simulink model "projsim"  (R2016a)
settings: Solver=VariableStepAuto  StartTime=0.0  StopTime=t_end  MaxStep=1/(w_e*50)  RelTol=1e-3
values from neighbouring files (symbols this model uses):
  bw_tot = 0.2    [cod.m]
  Csr = (Ls*Lr)/((Ls*Lr)-M^2)    (= 22.6278248588)    [cod.m]
  H_tot = 1.6    [cod.m]
  K_i = 0    [cod.m]
  K_p = 1    [cod.m]
  kt_l = 0    [cod.m]
  Lr = M+.0008    (= 0.0358)    [cod.m]
  Ls = M+.0008    (= 0.0358)    [cod.m]
  M = .035    (= 0.035)    [cod.m]
  P = 4    [cod.m]
  Rr = .1    (= 0.1)    [cod.m]
  Rs = .1    (= 0.1)    [cod.m]
  V_bus = 500    [cod.m]
  w_e_command = 2*pi*60    (= 376.991118431)    [cod.m]
settings Model: Creator=JSD5266  LastModifiedBy=Seth Barger

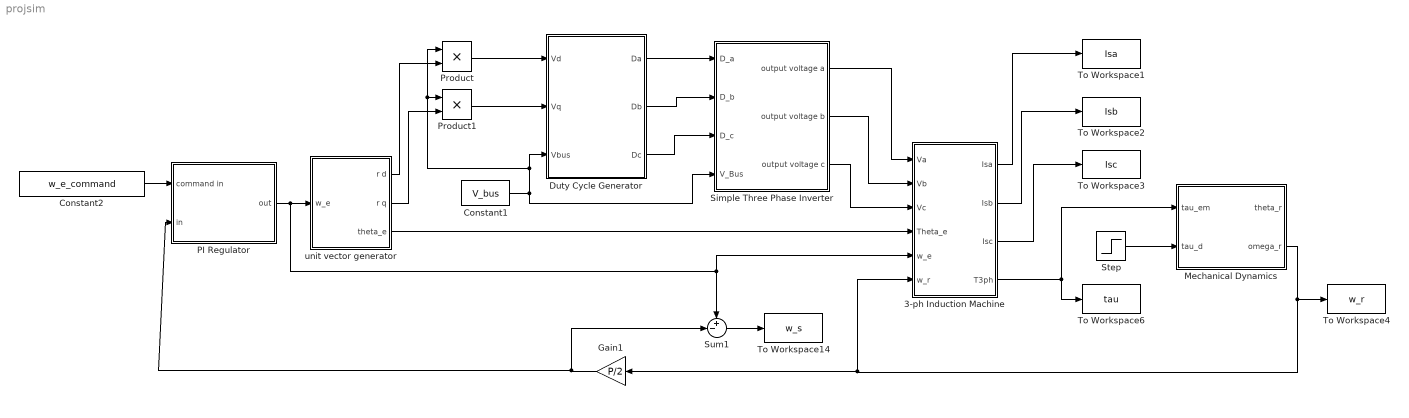
== system projsim ==
  3-ph Induction Machine : Subsystem
  Constant1 : Constant  Value=V_bus
  Constant2 : Constant  Value=w_e_command
  Duty Cycle Generator : Subsystem
  Gain1 : Gain  Gain=P/2
  Mechanical Dynamics : Subsystem
  PI Regulator : Subsystem
  Product : Product
  Product1 : Product
  Simple Three Phase Inverter : Subsystem
  Step : Step  Time=3  After=200  SampleTime=0
  Sum1 : Sum  Inputs=+-|
  To Workspace1 : ToWorkspace  VariableName=Isa  SampleTime=-1
  To Workspace14 : ToWorkspace  VariableName=w_s  SampleTime=-1
  To Workspace2 : ToWorkspace  VariableName=Isb  SampleTime=-1
  To Workspace3 : ToWorkspace  VariableName=Isc  SampleTime=-1
  To Workspace4 : ToWorkspace  VariableName=w_r  SampleTime=-1
  To Workspace6 : ToWorkspace  VariableName=tau  SampleTime=-1
  unit vector generator : Subsystem
  wires:
  3-ph Induction Machine/4(T3ph) -> To Workspace6/1, Mechanical Dynamics/1(tau_em)
  unit vector generator/3(theta_e) -> 3-ph Induction Machine/4(Theta_e)
  Step/1 -> Mechanical Dynamics/2(tau_d)
  Sum1/1 -> To Workspace14/1
  Gain1/1 -> PI Regulator/2(in), Sum1/2
  Simple Three Phase Inverter/3(output voltage c) -> 3-ph Induction Machine/3(Vc)
  Simple Three Phase Inverter/2(output voltage b) -> 3-ph Induction Machine/2(Vb)
  Simple Three Phase Inverter/1(output voltage a) -> 3-ph Induction Machine/1(Va)
  Duty Cycle Generator/1(Da) -> Simple Three Phase Inverter/1(D_a)
  Duty Cycle Generator/2(Db) -> Simple Three Phase Inverter/2(D_b)
  Duty Cycle Generator/3(Dc) -> Simple Three Phase Inverter/3(D_c)
  Constant1/1 -> Product1/1, Product/1, Duty Cycle Generator/3(Vbus), Simple Three Phase Inverter/4(V_Bus)
  Product/1 -> Duty Cycle Generator/1(Vd)
  unit vector generator/1(r d) -> Product/2
  Product1/1 -> Duty Cycle Generator/2(Vq)
  unit vector generator/2(r q) -> Product1/2
  Mechanical Dynamics/2(omega_r) -> To Workspace4/1, 3-ph Induction Machine/6(w_r), Gain1/1
  PI Regulator/1(out) -> Sum1/1, 3-ph Induction Machine/5(w_e), unit vector generator/1(w_e)
  Constant2/1 -> PI Regulator/1(command in)
  3-ph Induction Machine/1(Isa) -> To Workspace1/1
  3-ph Induction Machine/2(Isb) -> To Workspace2/1
  3-ph Induction Machine/3(Isc) -> To Workspace3/1

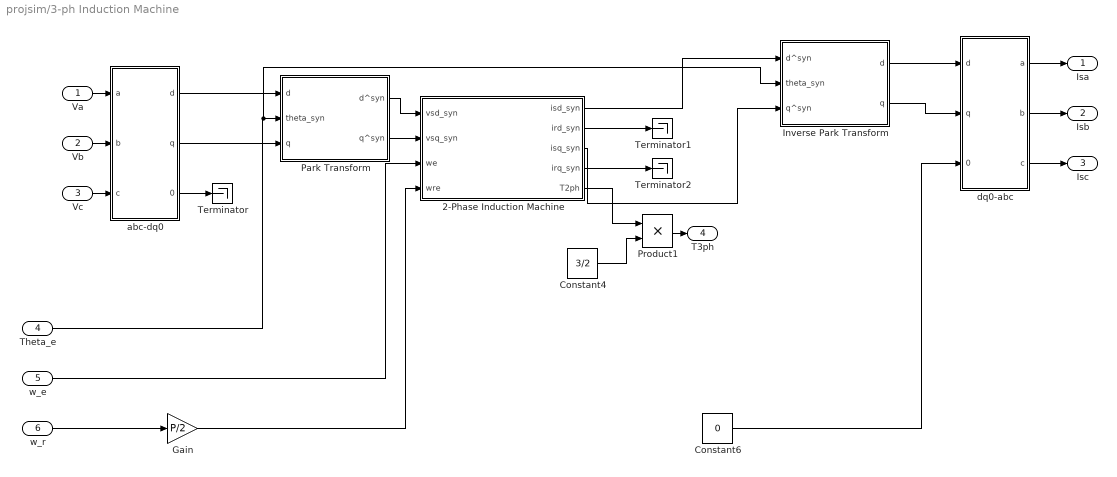
== system projsim/3-ph Induction Machine ==
  Va : Inport
  Vb : Inport  Port=2
  Vc : Inport  Port=3
  Theta_e : Inport  Port=4
  w_e : Inport  Port=5
  w_r : Inport  Port=6
  2-Phase Induction Machine : Subsystem
  Constant4 : Constant  Value=3/2
  Constant6 : Constant  Value=0
  Gain : Gain  Gain=P/2
  Inverse Park Transform : Subsystem
  Park Transform : Subsystem
  Product1 : Product
  Terminator : Terminator
  Terminator1 : Terminator
  Terminator2 : Terminator
  abc-dq0 : Subsystem
  dq0-abc : Subsystem
  Isa : Outport
  Isb : Outport  Port=2
  Isc : Outport  Port=3
  T3ph : Outport  Port=4
  wires:
  2-Phase Induction Machine/5(T2ph) -> Product1/1
  Constant4/1 -> Product1/2
  abc-dq0/3(0) -> Terminator/1
  Constant6/1 -> dq0-abc/3(0)
  Vc/1 -> abc-dq0/3(c)
  Vb/1 -> abc-dq0/2(b)
  Va/1 -> abc-dq0/1(a)
  dq0-abc/3(c) -> Isc/1
  dq0-abc/2(b) -> Isb/1
  dq0-abc/1(a) -> Isa/1
  Product1/1 -> T3ph/1
  2-Phase Induction Machine/2(ird_syn) -> Terminator1/1
  2-Phase Induction Machine/4(irq_syn) -> Terminator2/1
  Inverse Park Transform/1(d) -> dq0-abc/1(d)
  Inverse Park Transform/2(q) -> dq0-abc/2(q)
  2-Phase Induction Machine/1(isd_syn) -> Inverse Park Transform/1(d^syn)
  2-Phase Induction Machine/3(isq_syn) -> Inverse Park Transform/3(q^syn)
  abc-dq0/1(d) -> Park Transform/1(d)
  abc-dq0/2(q) -> Park Transform/3(q)
  Park Transform/1(d^syn) -> 2-Phase Induction Machine/1(vsd_syn)
  Park Transform/2(q^syn) -> 2-Phase Induction Machine/2(vsq_syn)
  Theta_e/1 -> Inverse Park Transform/2(theta_syn), Park Transform/2(theta_syn)
  w_e/1 -> 2-Phase Induction Machine/3(we)
  w_r/1 -> Gain/1
  Gain/1 -> 2-Phase Induction Machine/4(wre)

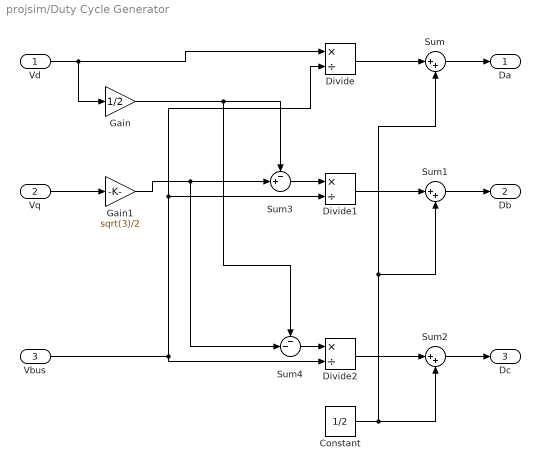
== system projsim/Duty Cycle Generator ==
  Vd : Inport
  Vq : Inport  Port=2
  Vbus : Inport  Port=3
  Constant : Constant  Value=1/2
  Divide : Product  Inputs=*/
  Divide1 : Product  Inputs=*/
  Divide2 : Product  Inputs=*/
  Gain : Gain  Gain=1/2
  Gain1 : Gain  Gain=sqrt(3)/2
  Sum : Sum  Inputs=|++
  Sum1 : Sum  Inputs=|++
  Sum2 : Sum  Inputs=|++
  Sum3 : Sum  Inputs=-+|
  Sum4 : Sum  Inputs=--|
  Da : Outport
  Db : Outport  Port=2
  Dc : Outport  Port=3
  wires:
  Sum2/1 -> Dc/1
  Constant/1 -> Sum2/2, Sum1/2, Sum/2
  Vd/1 -> Gain/1, Divide/1
  Sum/1 -> Da/1
  Divide1/1 -> Sum1/1
  Sum1/1 -> Db/1
  Vbus/1 -> Divide1/2, Divide/2, Divide2/2
  Vq/1 -> Gain1/1
  Sum3/1 -> Divide1/1
  Gain1/1 -> Sum4/2, Sum3/2
  Sum4/1 -> Divide2/1
  Divide/1 -> Sum/1
  Divide2/1 -> Sum2/1
  Gain/1 -> Sum4/1, Sum3/1

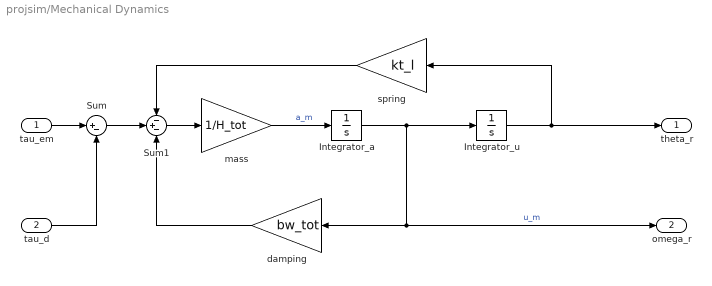
== system projsim/Mechanical Dynamics ==
  tau_em : Inport
  tau_d : Inport  Port=2
  Integrator_a : Integrator
  Integrator_u : Integrator
  Sum : Sum  Inputs=|+-
  Sum1 : Sum  Inputs=-+-
  damping : Gain  Gain=bw_tot
  mass : Gain  Gain=1/H_tot
  spring : Gain  Gain=kt_l
  theta_r : Outport
  omega_r : Outport  Port=2
  wires:
  tau_em/1 -> Sum/1
  tau_d/1 -> Sum/2
  mass/1 -> Integrator_a/1  "a_m"
  Integrator_a/1 -> Integrator_u/1, omega_r/1, damping/1  "u_m"
  Integrator_u/1 -> theta_r/1, spring/1
  Sum/1 -> Sum1/2
  Sum1/1 -> mass/1
  damping/1 -> Sum1/3
  spring/1 -> Sum1/1

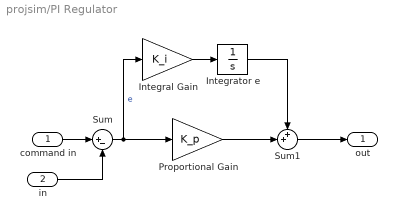
== system projsim/PI Regulator ==
  command in : Inport
  in : Inport  Port=2
  Integral Gain : Gain  Gain=K_i  SaturateOnIntegerOverflow=on  OutDataTypeStr=Inherit: Same as input  ParamDataTypeStr=Inherit: Same as input
  Integrator e : Integrator
  Proportional Gain : Gain  Gain=K_p  SaturateOnIntegerOverflow=on  OutDataTypeStr=Inherit: Same as input  ParamDataTypeStr=Inherit: Same as input
  Sum : Sum  Inputs=|+-  SaturateOnIntegerOverflow=on
  Sum1 : Sum  Inputs=++|  SaturateOnIntegerOverflow=on
  out : Outport
  wires:
  Sum/1 -> Integral Gain/1, Proportional Gain/1  "e"
  command in/1 -> Sum/1
  in/1 -> Sum/2
  Proportional Gain/1 -> Sum1/2
  Sum1/1 -> out/1
  Integral Gain/1 -> Integrator e/1
  Integrator e/1 -> Sum1/1

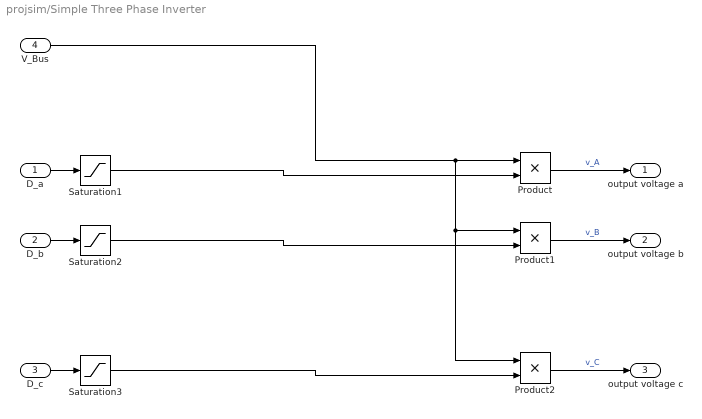
== system projsim/Simple Three Phase Inverter ==
  D_a : Inport
  D_b : Inport  Port=2
  D_c : Inport  Port=3
  V_Bus : Inport  Port=4
  Product : Product
  Product1 : Product
  Product2 : Product
  Saturation1 : Saturate  UpperLimit=1  LowerLimit=0
  Saturation2 : Saturate  UpperLimit=1  LowerLimit=0
  Saturation3 : Saturate  UpperLimit=1  LowerLimit=0
  output voltage a : Outport
  output voltage b : Outport  Port=2
  output voltage c : Outport  Port=3
  wires:
  D_a/1 -> Saturation1/1
  D_b/1 -> Saturation2/1
  D_c/1 -> Saturation3/1
  Product/1 -> output voltage a/1  "v_A"
  Product2/1 -> output voltage c/1  "v_C"
  Product1/1 -> output voltage b/1  "v_B"
  V_Bus/1 -> Product2/1, Product1/1, Product/1
  Saturation1/1 -> Product/2
  Saturation2/1 -> Product1/2
  Saturation3/1 -> Product2/2

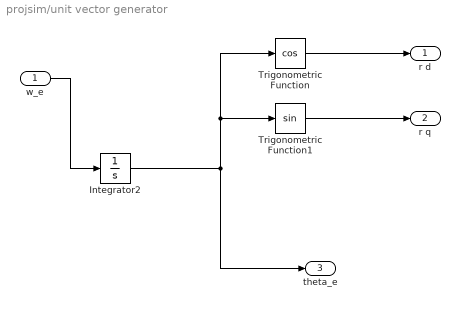
== system projsim/unit vector generator ==
  w_e : Inport
  Integrator2 : Integrator
  Trigonometric Function : Trigonometry  Operator=cos
  Trigonometric Function1 : Trigonometry
  r d : Outport
  r q : Outport  Port=2
  theta_e : Outport  Port=3
  wires:
  w_e/1 -> Integrator2/1
  Integrator2/1 -> Trigonometric Function1/1, Trigonometric Function/1, theta_e/1
  Trigonometric Function1/1 -> r q/1
  Trigonometric Function/1 -> r d/1

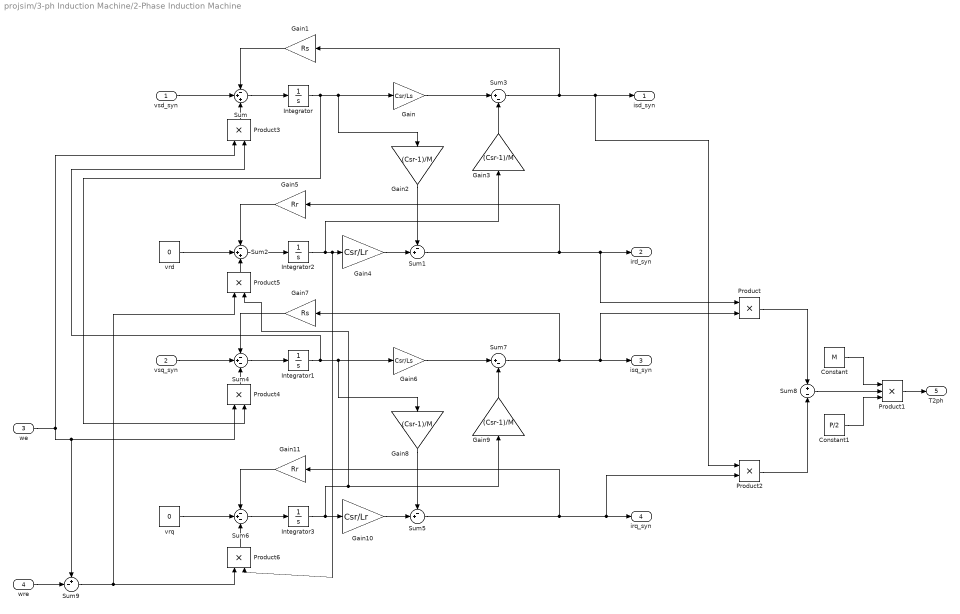
== system projsim/3-ph Induction Machine/2-Phase Induction Machine ==
  vsd_syn : Inport
  vsq_syn : Inport  Port=2
  we : Inport  Port=3
  wre : Inport  Port=4
  Constant : Constant  Value=M
  Constant1 : Constant  Value=P/2
  Gain : Gain  Gain=Csr/Ls
  Gain1 : Gain  Gain=Rs
  Gain10 : Gain  Gain=Csr/Lr
  Gain11 : Gain  Gain=Rr
  Gain{2..3,8..9} (4 alike) : Gain  Gain=(Csr-1)/M
  Gain4 : Gain  Gain=Csr/Lr
  Gain5 : Gain  Gain=Rr
  Gain6 : Gain  Gain=Csr/Ls
  Gain7 : Gain  Gain=Rs
  Integrator{,1..3} (4 alike) : Integrator
  Product{,2..6} (6 alike) : Product
  Product1 : Product  Inputs=3
  Sum : Sum  Inputs=-++
  Sum1 : Sum  Inputs=-+|
  Sum2 : Sum  Inputs=-++
  Sum3 : Sum  Inputs=|+-
  Sum4 : Sum  Inputs=-+-
  Sum5 : Sum  Inputs=-+|
  Sum6 : Sum  Inputs=-+-
  Sum7 : Sum  Inputs=|+-
  Sum8 : Sum  Inputs=+-
  Sum9 : Sum  Inputs=+-|
  vrd : Constant  Value=0
  vrq : Constant  Value=0
  isd_syn : Outport
  ird_syn : Outport  Port=2
  isq_syn : Outport  Port=3
  irq_syn : Outport  Port=4
  T2ph : Outport  Port=5
  wires:
  Product2/1 -> Sum8/2
  Constant1/1 -> Product1/3
  Sum3/1 -> isd_syn/1, Product2/1, Gain1/1
  Product1/1 -> T2ph/1
  Sum8/1 -> Product1/2
  Constant/1 -> Product1/1
  Product/1 -> Sum8/1
  Gain5/1 -> Sum2/1
  Sum1/1 -> Gain5/1, ird_syn/1, Product/1
  Sum2/1 -> Integrator2/1
  vrd/1 -> Sum2/2
  Integrator2/1 -> Gain3/1, Product6/2, Gain4/1
  Sum/1 -> Integrator/1
  Integrator/1 -> Gain/1, Gain2/1, Product4/2
  vsd_syn/1 -> Sum/2
  Gain3/1 -> Sum3/2
  Gain1/1 -> Sum/1
  Sum4/1 -> Integrator1/1
  Gain8/1 -> Sum5/1
  Sum6/1 -> Integrator3/1
  Gain/1 -> Sum3/1
  vrq/1 -> Sum6/2
  Gain6/1 -> Sum7/1
  Gain10/1 -> Sum5/2
  Gain11/1 -> Sum6/1
  Gain9/1 -> Sum7/2
  Gain7/1 -> Sum4/1
  vsq_syn/1 -> Sum4/2
  Integrator3/1 -> Gain10/1, Gain9/1, Product5/2
  Gain4/1 -> Sum1/2
  Sum7/1 -> Gain7/1, isq_syn/1, Product/2
  Integrator1/1 -> Product3/2, Gain8/1, Gain6/1
  Sum5/1 -> irq_syn/1, Product2/2, Gain11/1
  Gain2/1 -> Sum1/1
  Product3/1 -> Sum/3
  Product4/1 -> Sum4/3
  we/1 -> Product3/1, Sum9/1, Product4/1
  Product5/1 -> Sum2/3
  Product6/1 -> Sum6/3
  wre/1 -> Sum9/2
  Sum9/1 -> Product5/1, Product6/1

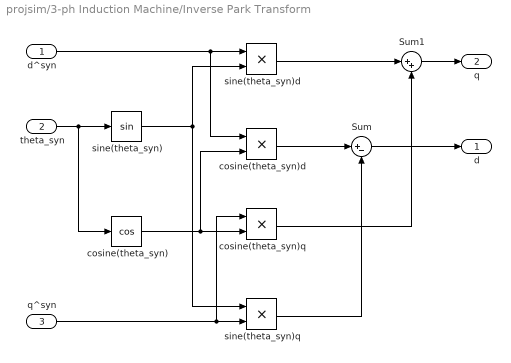
== system projsim/3-ph Induction Machine/Inverse Park Transform ==
  d^syn : Inport
  theta_syn : Inport  Port=2
  q^syn : Inport  Port=3
  Sum : Sum  Inputs=|+-
  Sum1 : Sum  Inputs=|++
  cosine(theta_syn) : Trigonometry  Operator=cos
  cosine(theta_syn)d : Product
  cosine(theta_syn)q : Product
  sine(theta_syn) : Trigonometry
  sine(theta_syn)d : Product
  sine(theta_syn)q : Product
  d : Outport
  q : Outport  Port=2
  wires:
  Sum1/1 -> q/1
  cosine(theta_syn)q/1 -> Sum1/2
  cosine(theta_syn)d/1 -> Sum/1
  q^syn/1 -> cosine(theta_syn)q/1, sine(theta_syn)q/2
  sine(theta_syn)q/1 -> Sum/2
  cosine(theta_syn)/1 -> cosine(theta_syn)q/2, cosine(theta_syn)d/2
  Sum/1 -> d/1
  sine(theta_syn)d/1 -> Sum1/1
  theta_syn/1 -> cosine(theta_syn)/1, sine(theta_syn)/1
  d^syn/1 -> cosine(theta_syn)d/1, sine(theta_syn)d/1
  sine(theta_syn)/1 -> sine(theta_syn)q/1, sine(theta_syn)d/2

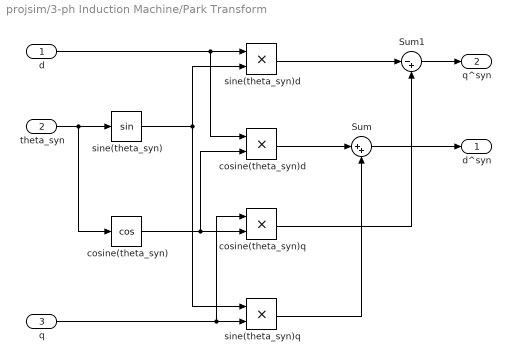
== system projsim/3-ph Induction Machine/Park Transform ==
  d : Inport
  theta_syn : Inport  Port=2
  q : Inport  Port=3
  Sum : Sum  Inputs=|++
  Sum1 : Sum  Inputs=|-+
  cosine(theta_syn) : Trigonometry  Operator=cos
  cosine(theta_syn)d : Product
  cosine(theta_syn)q : Product
  sine(theta_syn) : Trigonometry
  sine(theta_syn)d : Product
  sine(theta_syn)q : Product
  d^syn : Outport
  q^syn : Outport  Port=2
  wires:
  Sum1/1 -> q^syn/1
  cosine(theta_syn)q/1 -> Sum1/2
  cosine(theta_syn)d/1 -> Sum/1
  q/1 -> cosine(theta_syn)q/1, sine(theta_syn)q/2
  sine(theta_syn)q/1 -> Sum/2
  cosine(theta_syn)/1 -> cosine(theta_syn)q/2, cosine(theta_syn)d/2
  Sum/1 -> d^syn/1
  sine(theta_syn)d/1 -> Sum1/1
  theta_syn/1 -> cosine(theta_syn)/1, sine(theta_syn)/1
  d/1 -> cosine(theta_syn)d/1, sine(theta_syn)d/1
  sine(theta_syn)/1 -> sine(theta_syn)q/1, sine(theta_syn)d/2

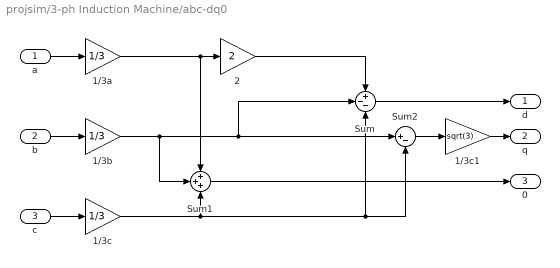
== system projsim/3-ph Induction Machine/abc-dq0 ==
  a : Inport
  b : Inport  Port=2
  c : Inport  Port=3
  1/3a : Gain  Gain=1/3
  1/3b : Gain  Gain=1/3
  1/3c : Gain  Gain=1/3
  1/3c1 : Gain  Gain=sqrt(3)
  2 : Gain  Gain=2
  Sum : Sum  Inputs=+--
  Sum1 : Sum  Inputs=+++
  Sum2 : Sum  Inputs=|+-
  d : Outport
  q : Outport  Port=2
  0 : Outport  Port=3
  wires:
  c/1 -> 1/3c/1
  b/1 -> 1/3b/1
  a/1 -> 1/3a/1
  1/3a/1 -> Sum1/1, 2/1
  2/1 -> Sum/1
  1/3b/1 -> Sum1/2, Sum2/1, Sum/2
  Sum/1 -> d/1
  1/3c/1 -> Sum1/3, Sum2/2, Sum/3
  Sum1/1 -> 0/1
  Sum2/1 -> 1/3c1/1
  1/3c1/1 -> q/1

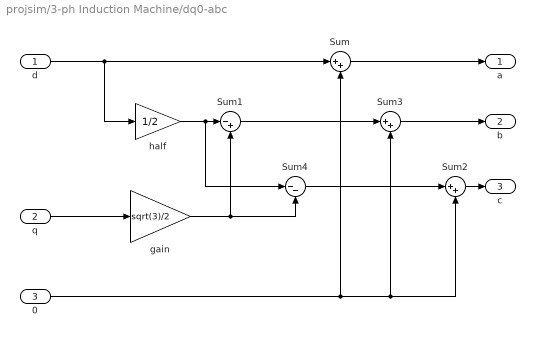
== system projsim/3-ph Induction Machine/dq0-abc ==
  d : Inport
  q : Inport  Port=2
  0 : Inport  Port=3
  Sum : Sum  Inputs=|++
  Sum1 : Sum  Inputs=|-+
  Sum2 : Sum  Inputs=|++
  Sum3 : Sum  Inputs=|++
  Sum4 : Sum  Inputs=|--
  gain : Gain  Gain=sqrt(3)/2
  half : Gain  Gain=1/2
  a : Outport
  b : Outport  Port=2
  c : Outport  Port=3
  wires:
  Sum/1 -> a/1
  d/1 -> half/1, Sum/1
  Sum1/1 -> Sum3/1
  0/1 -> Sum/2, Sum2/2, Sum3/2
  q/1 -> gain/1
  gain/1 -> Sum4/2, Sum1/2
  Sum2/1 -> c/1
  Sum3/1 -> b/1
  half/1 -> Sum4/1, Sum1/1
  Sum4/1 -> Sum2/1
